simulink model "pendSimQController"  (R2024a)
settings: Solver=FixedStepAuto  StartTime=0.0  StopTime=5  FixedStep=0.005  MaxStep=0.001  RelTol=1e-3
settings Model: Creator=mattf  LastModifiedBy=ariellevy

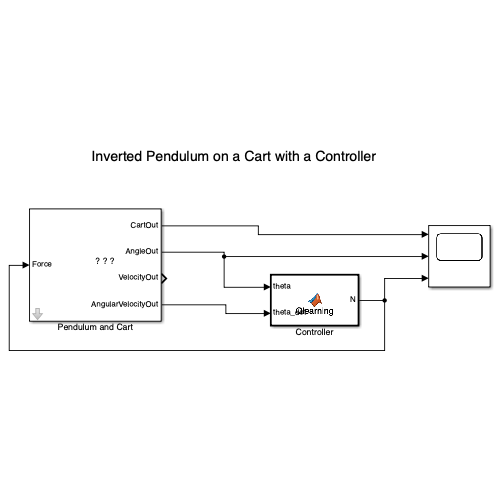
[thumbnail: Simulink's stored preview of the top-level diagram]
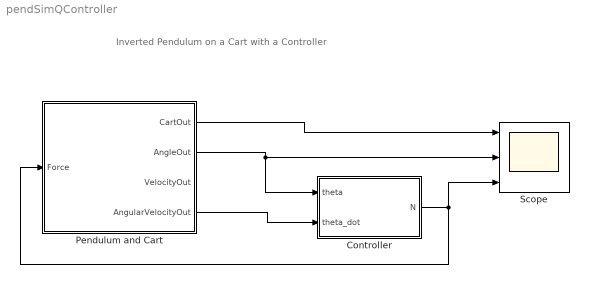
== system pendSimQController ==
  note: Inverted Pendulum on a Cart with a Controller
  Controller : MATLAB Function  TreatAsAtomicUnit=on  SystemSampleTime=0.005
  Pendulum and Cart : Subsystem  mask{Mcart=0.5, m=0.2, l=0.3/2, g=9.8, init=0.07}
      mask prompts: Mcart "Cart Mass (kg):"; m "Pend Mass (kg):"; l "COM Distance (m):"; g "Acc due to Gravity (g):"; init "Initial Angle (rad):"
      mask Display: image('pen img.png');
  Scope : Scope  NumInputPorts=3
  wires:
  Pendulum and Cart/2(AngleOut) -> Controller/1(theta), Scope/2
  Controller/1(N) -> Scope/3, Pendulum and Cart/1(Force)
  Pendulum and Cart/1(CartOut) -> Scope/1
  Pendulum and Cart/4(AngularVelocityOut) -> Controller/2(theta_dot)

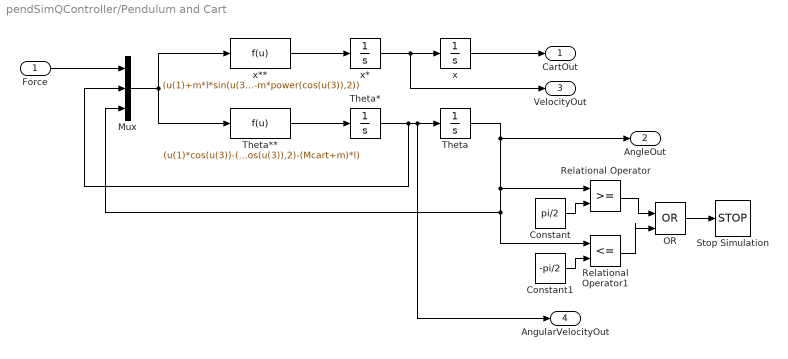
== system pendSimQController/Pendulum and Cart ==
  Force : Inport
  Constant : Constant  Value=pi/2
  Constant1 : Constant  Value=-pi/2
  Mux : Mux  Inputs=3
  OR : Logic  Operator=OR  IconShape=distinctive  AllPortsSameDT=off  OutDataTypeStr=boolean
  Relational Operator : RelationalOperator  OutDataTypeStr=boolean  RndMeth=Simplest  InputSameDT=off
  Relational Operator1 : RelationalOperator  Operator=<=  OutDataTypeStr=boolean  RndMeth=Simplest  InputSameDT=off
  Stop Simulation : Stop
  Theta : Integrator  InitialCondition=init
  Theta* : Integrator
  Theta** : Fcn  Expr=(u(1)*cos(u(3))-(Mcart+m)*g*sin(u(3))+m*l*cos(u(3))*sin(u(3))*power(u(2),2))/(m*l*power(cos(u(3)),2)-(Mcart+m)*l)
  x : Integrator
  x* : Integrator
  x** : Fcn  Expr=(u(1)+m*l*sin(u(3))*power(u(2),2)-m*g*cos(u(3))*sin(u(3)))/(Mcart+m-m*power(cos(u(3)),2))
  CartOut : Outport
  AngleOut : Outport  Port=2
  VelocityOut : Outport  Port=3
  AngularVelocityOut : Outport  Port=4
  wires:
  Mux/1 -> x**/1, Theta**/1
  x/1 -> CartOut/1
  Force/1 -> Mux/1
  Theta**/1 -> Theta*/1
  x**/1 -> x*/1
  Theta/1 -> AngleOut/1, Relational Operator1/1, Mux/3, Relational Operator/1
  x*/1 -> VelocityOut/1, x/1
  Theta*/1 -> Mux/2, AngularVelocityOut/1, Theta/1
  Constant/1 -> Relational Operator/2
  OR/1 -> Stop Simulation/1
  Relational Operator1/1 -> OR/2
  Constant1/1 -> Relational Operator1/2
  Relational Operator/1 -> OR/1

== matlab function pendSimQController/Controller ==
  settings: updateMethod=DISCRETE
  data: N output; theta input; theta_dot input
function N = Qlearning(theta, theta_dot)

    % call extrinsic python function
    coder.extrinsic('py.QLearningController.controller_call');

    % Call Python function and return result
    N = coder.nullcopy(zeros(1,1)); % no clue why, but this is need.
    N = double(py.QLearningController.controller_call(theta, theta_dot));
    end
